simulink model "AAI"  (R2020a)
settings: Solver=FixedStepAuto  StartTime=0.0  StopTime=10.0  FixedStep=1e-3  RelTol=1e-3  EnableMultiTasking=on
undefined symbols (not defined in the file or in its folder): D0, D1, D10, D11, D12, D13, D2, D3, D4, D5, D6, D7, D8, D9, PTA0, PTA1, PTA2, PTB23, PTB9, PTC16, PTC17, PTC2, PTC3, PTC4, PTD0, PTD1, PTD2, PTD3
libraries: frdmk64flib x15
settings Model: ExtModeTrigDuration=5  Creator=davidmercuri  LastModifiedBy=davidmercuri
settings OptimizationCC: EnhancedBackFolding=on  PassReuseOutputArgsAs=Individual arguments  ZeroExternalMemoryAtStartup=off  ZeroInternalMemoryAtStartup=off  MaxStackSize=64  OptimizeBlockOrder=speed  DifferentSizesBufferReuse=on  OptimizationCustomize=off  EfficientTunableParamExpr=on
settings DebuggingCC: ParameterTunabilityLossMsg=error
settings HardwareCC: ProdBitPerPointer=32  ProdBitPerSizeT=32  ProdBitPerPtrDiffT=32  ProdLargestAtomicInteger=Long  ProdLargestAtomicFloat=Double  ProdWordSize=32  ProdHWDeviceType=ARM Compatible->ARM Cortex
settings SFSimCC: MATLABDynamicMemAlloc=off
settings RTWCC: SystemTargetFile=ert.tlc  HardwareBoard=NXP FRDM-K64F  TemplateMakefile=ert_default_tmf  Toolchain=GNU Tools for ARM Embedded Processors
settings CodeAppCC: ForceParamTrailComments=on  IgnoreCustomStorageClasses=off  OperatorAnnotations=on  SimulinkDataObjDesc=on  SFDataObjDesc=on  InsertBlockDesc=on

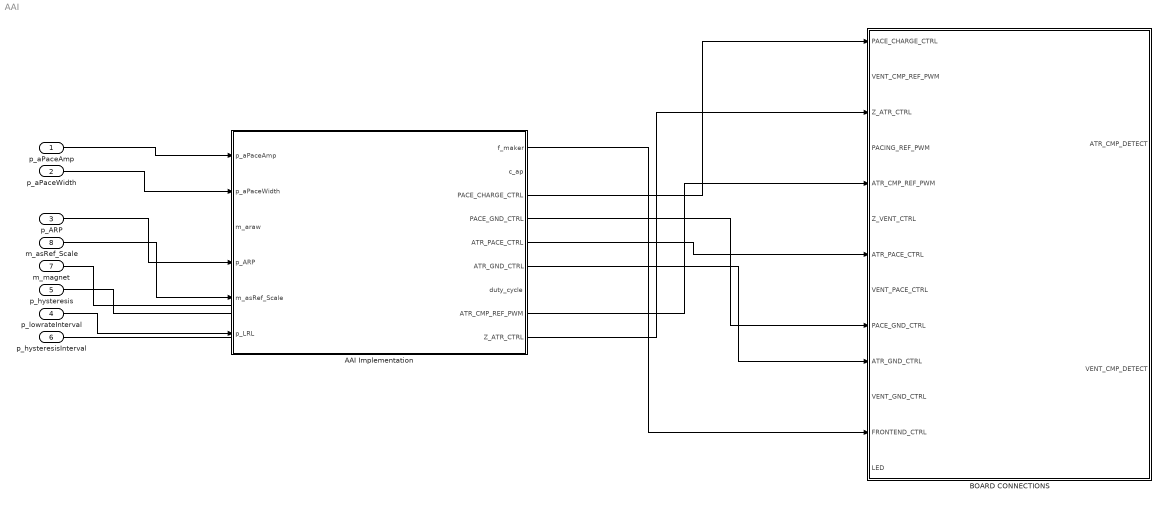
== system AAI ==
  p_aPaceAmp : Inport
  p_aPaceWidth : Inport  Port=2
  p_ARP : Inport  Port=3
  p_lowrateInterval : Inport  Port=4
  p_hysteresis : Inport  Port=5
  p_hysteresisInterval : Inport  Port=6
  m_magnet : Inport  Port=7
  m_asRef_Scale : Inport  Port=8
  AAI Implementation : Subsystem
  BOARD CONNECTIONS : Subsystem
  wires:
  p_aPaceAmp/1 -> AAI Implementation/1(p_aPaceAmp)
  p_lowrateInterval/1 -> AAI Implementation/6(p_LRL)
  p_hysteresisInterval/1 -> ?
  p_ARP/1 -> AAI Implementation/4(p_ARP)
  p_aPaceWidth/1 -> AAI Implementation/2(p_aPaceWidth)
  m_asRef_Scale/1 -> AAI Implementation/5(m_asRef_Scale)
  m_magnet/1 -> ?
  p_hysteresis/1 -> ?
  AAI Implementation/3(PACE_CHARGE_CTRL) -> BOARD CONNECTIONS/1(PACE_CHARGE_CTRL)
  AAI Implementation/8(ATR_CMP_REF_PWM) -> BOARD CONNECTIONS/5(ATR_CMP_REF_PWM)
  AAI Implementation/5(ATR_PACE_CTRL) -> BOARD CONNECTIONS/7(ATR_PACE_CTRL)
  AAI Implementation/4(PACE_GND_CTRL) -> BOARD CONNECTIONS/9(PACE_GND_CTRL)
  AAI Implementation/6(ATR_GND_CTRL) -> BOARD CONNECTIONS/10(ATR_GND_CTRL)
  AAI Implementation/1(f_maker) -> BOARD CONNECTIONS/12(FRONTEND_CTRL)
  AAI Implementation/9(Z_ATR_CTRL) -> BOARD CONNECTIONS/3(Z_ATR_CTRL)

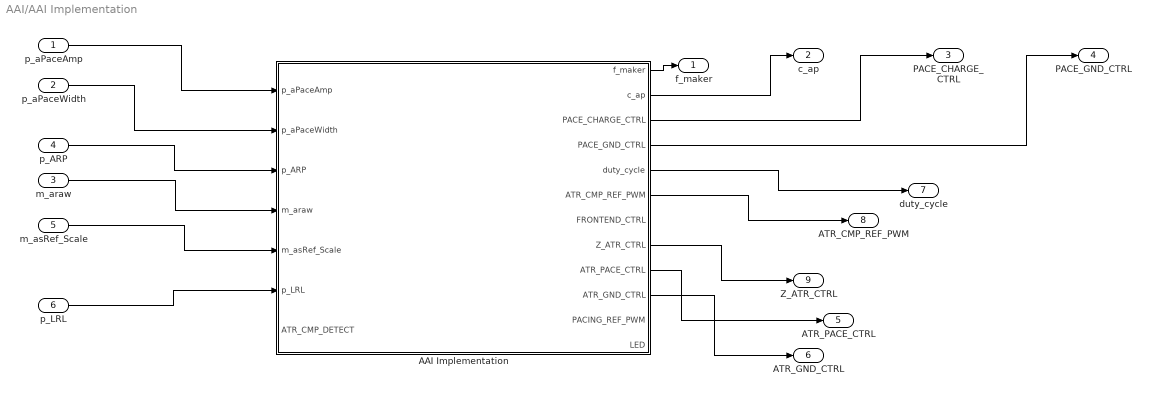
== system AAI/AAI Implementation ==
  p_aPaceAmp : Inport
  p_aPaceWidth : Inport  Port=2
  m_araw : Inport  Port=3
  p_ARP : Inport  Port=4
  m_asRef_Scale : Inport  Port=5
  p_LRL : Inport  Port=6
  AAI Implementation : Stateflow chart  TreatAsAtomicUnit=on
  f_maker : Outport
  c_ap : Outport  Port=2
  PACE_CHARGE_CTRL : Outport  Port=3
  PACE_GND_CTRL : Outport  Port=4
  ATR_PACE_CTRL : Outport  Port=5
  ATR_GND_CTRL : Outport  Port=6
  duty_cycle : Outport  Port=7
  ATR_CMP_REF_PWM : Outport  Port=8
  Z_ATR_CTRL : Outport  Port=9
  wires:
  m_asRef_Scale/1 -> AAI Implementation/5(m_asRef_Scale)
  AAI Implementation/6(ATR_CMP_REF_PWM) -> ATR_CMP_REF_PWM/1
  AAI Implementation/1(f_maker) -> f_maker/1
  AAI Implementation/2(c_ap) -> c_ap/1
  AAI Implementation/5(duty_cycle) -> duty_cycle/1
  p_aPaceWidth/1 -> AAI Implementation/2(p_aPaceWidth)
  AAI Implementation/3(PACE_CHARGE_CTRL) -> PACE_CHARGE_CTRL/1
  m_araw/1 -> AAI Implementation/4(m_araw)
  AAI Implementation/4(PACE_GND_CTRL) -> PACE_GND_CTRL/1
  p_LRL/1 -> AAI Implementation/6(p_LRL)
  p_aPaceAmp/1 -> AAI Implementation/1(p_aPaceAmp)
  p_ARP/1 -> AAI Implementation/3(p_ARP)
  AAI Implementation/10(ATR_GND_CTRL) -> ATR_GND_CTRL/1
  AAI Implementation/9(ATR_PACE_CTRL) -> ATR_PACE_CTRL/1
  AAI Implementation/8(Z_ATR_CTRL) -> Z_ATR_CTRL/1

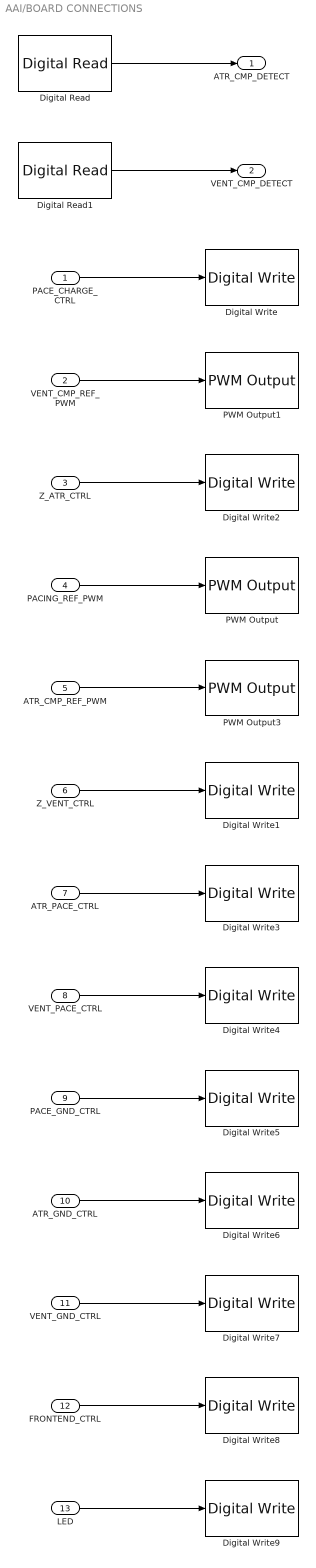
== system AAI/BOARD CONNECTIONS ==
  PACE_CHARGE_CTRL : Inport
  VENT_CMP_REF_PWM : Inport  Port=2
  Z_ATR_CTRL : Inport  Port=3
  PACING_REF_PWM : Inport  Port=4
  ATR_CMP_REF_PWM : Inport  Port=5
  Z_VENT_CTRL : Inport  Port=6
  ATR_PACE_CTRL : Inport  Port=7
  VENT_PACE_CTRL : Inport  Port=8
  PACE_GND_CTRL : Inport  Port=9
  ATR_GND_CTRL : Inport  Port=10
  VENT_GND_CTRL : Inport  Port=11
  FRONTEND_CTRL : Inport  Port=12
  LED : Inport  Port=13
  Digital Read : frdmk64flib/Digital Read  Whichpin=PTC16 (D0)  SampleTime=-1
  Digital Read1 : frdmk64flib/Digital Read  Whichpin=PTC17 (D1)  SampleTime=-1
  Digital Write : frdmk64flib/Digital Write  Whichpin=PTB9 (D2)
  Digital Write1 : frdmk64flib/Digital Write  Whichpin=PTC3 (D7)
  Digital Write2 : frdmk64flib/Digital Write  Whichpin=PTB23 (D4)
  Digital Write3 : frdmk64flib/Digital Write  Whichpin=PTA0 (D8)
  Digital Write4 : frdmk64flib/Digital Write  Whichpin=PTC4 (D9)
  Digital Write5 : frdmk64flib/Digital Write  Whichpin=PTD0 (D10)
  Digital Write6 : frdmk64flib/Digital Write  Whichpin=PTD2 (D11)
  Digital Write7 : frdmk64flib/Digital Write  Whichpin=PTD3 (D12)
  Digital Write8 : frdmk64flib/Digital Write  Whichpin=PTD1 (D13)
  Digital Write9 : frdmk64flib/Digital Write  Whichpin=RED_LED
  PWM Output : frdmk64flib/PWM Output  Whichpin=PTA2 (D5)  InitialFrequency=2000  InitialDutyCycle=0
  PWM Output1 : frdmk64flib/PWM Output  Whichpin=PTA1 (D3)  InitialFrequency=2000  InitialDutyCycle=0
  PWM Output3 : frdmk64flib/PWM Output  Whichpin=PTC2 (D6)  InitialFrequency=2000  InitialDutyCycle=100
  ATR_CMP_DETECT : Outport
  VENT_CMP_DETECT : Outport  Port=2
  wires:
  Digital Read/1 -> ATR_CMP_DETECT/1
  Digital Read1/1 -> VENT_CMP_DETECT/1
  VENT_CMP_REF_PWM/1 -> PWM Output1/1
  PACE_CHARGE_CTRL/1 -> Digital Write/1
  Z_ATR_CTRL/1 -> Digital Write2/1
  PACING_REF_PWM/1 -> PWM Output/1
  ATR_CMP_REF_PWM/1 -> PWM Output3/1
  Z_VENT_CTRL/1 -> Digital Write1/1
  ATR_PACE_CTRL/1 -> Digital Write3/1
  VENT_PACE_CTRL/1 -> Digital Write4/1
  PACE_GND_CTRL/1 -> Digital Write5/1
  ATR_GND_CTRL/1 -> Digital Write6/1
  VENT_GND_CTRL/1 -> Digital Write7/1
  FRONTEND_CTRL/1 -> Digital Write8/1
  LED/1 -> Digital Write9/1

== stateflow chart AAI/AAI Implementation/AAI Implementation ==
  state AAI_PACING
    entry:
    FRONTEND_CTRL = false;
    %
    ATR_PACE_CTRL = true;
    PACE_CHARGE_CTRL = false
    %
    ATR_GND_CTRL = false;
    PACE_GND_CTRL = true;
    %
    Z_ATR_CTRL = false;
    LED = true;
  state AAI_SENSING
    entry:
    FRONTEND_CTRL = true;
    %
    ATR_PACE_CTRL = false;
    PACE_CHARGE_CTRL = true;
    %
    ATR_GND_CTRL = true;
    PACE_GND_CTRL = true;
    %
    Z_ATR_CTRL = false;
    %Double Check
    ATR_CMP_REF_PWM = m_asRef_Scale * m_araw;
    PACING_REF_PWM = p_aPaceAmp;
  state AAI_REFRACTORY
    entry:
    FRONTEND_CTRL = true;
    %
    PACE_CHARGE_CTRL = false;
    ATR_PACE_CTRL = false;
    %
    ATR_GND_CTRL = true;
    PACE_GND_CTRL = true;
  (default) -> AAI_SENSING
  AAI_SENSING -> AAI_PACING [order 1] : [after((60000/p_LRL-p_aPaceWidth), msec) && (ATR_CMP_DETECT == 0)]
  AAI_REFRACTORY -> AAI_SENSING : [after(p_ARP), msec]
  AAI_PACING -> AAI_REFRACTORY : [after(p_aPaceWidth, msec)]
  AAI_SENSING -> AAI_REFRACTORY [order 2] : [ATR_CMP_DETECT == 1]
  data: p_aPaceAmp input [500..7000]; p_aPaceWidth input double [0.1..1.9]; p_ARP input [150..500]; m_araw input double [5000.0..0.0]; m_asRef_Scale input boolean [0..1]; f_maker output; c_ap output; PACE_CHARGE_CTRL output boolean [0..1]; PACE_GND_CTRL output boolean [0..1]; duty_cycle output; ATR_CMP_REF_PWM output; FRONTEND_CTRL output boolean; Z_ATR_CTRL output boolean; ATR_PACE_CTRL output boolean; ATR_GND_CTRL output boolean; PACING_REF_PWM output; LED output; p_LRL input; ATR_CMP_DETECT input
